simulink model "cart_pole_model"  (R2020b)
settings: Solver=VariableStepAuto  StartTime=0.0  StopTime=10.0  RelTol=1e-3
undefined symbols (not defined in the file): b, D_theta, D_x, g, I, I_theta, I_x, l, m, M, P_theta, P_x
libraries: pid_lib x4
settings Model: Creator=Illia  LastModifiedBy=Illia

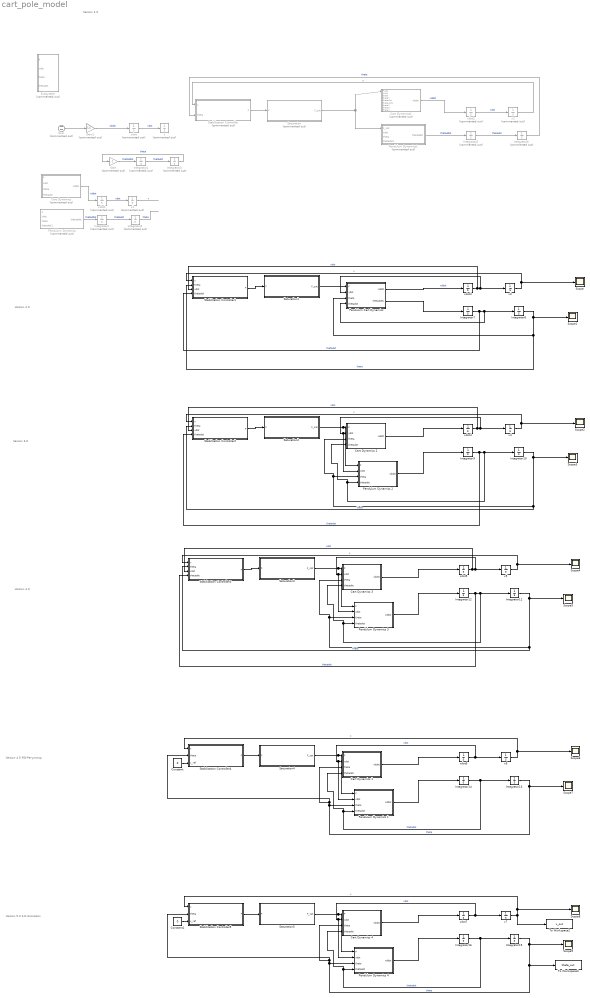
== system cart_pole_model ==
  note: Version 1.0
  note: Version 2.0
  note: Version 3.0
  note: Version 4.0
  note: Version 4.5
      | PID-Регулятор
  note: Version 5.0
      | 2-D Animation
  Cart Dynamics : Subsystem  Commented=on
  Cart Dynamics 1 : Subsystem
  Cart Dynamics 2 : Subsystem
  Cart Dynamics 3 : Subsystem
  Cart Dynamics 4 : Subsystem
  Cart Dynamics1 : Subsystem  Commented=on
  Constant : Constant  Value=0
  Constant1 : Constant  Value=0
  Gain : Gain  Commented=on  Gain=-1
  Gain1 : Gain  Commented=on  Gain=50
  Integrator{1..5} (5 alike) : Integrator  Commented=on
  Integrator{8,10..11,13,15} (5 alike) : Integrator  InitialCondition=0.1
  Integrator{7,9,12,14,16} (5 alike) : Integrator
  Integrator6 : Integrator  Commented=on  InitialCondition=0.1
  Pendulum Cart Dynamics : MATLAB Function  TreatAsAtomicUnit=on
  Pendulum Dynamics : Subsystem  Commented=on
  Pendulum Dynamics 1 : Subsystem
  Pendulum Dynamics 2 : Subsystem
  Pendulum Dynamics 3 : Subsystem
  Pendulum Dynamics 4 : Subsystem
  Pendulum Dynamics1 : Subsystem  Commented=on
  Saturation : Subsystem  Commented=on
  Saturation1 : Subsystem
  Saturation2 : Subsystem
  Saturation3 : Subsystem
  Saturation4 : Subsystem
  Saturation5 : Subsystem
  Scope{,1..9} (10 alike) : Scope
  Stabilization Controller : Subsystem  Commented=on
  Stabilization Controller1 : Subsystem
  Stabilization Controller2 : Subsystem
  Stabilization Controller3 : Subsystem
  Stabilization Controller4 : Subsystem
  Stabilization Controller5 : Subsystem
  Subsystem : Subsystem  Commented=on
  Sum : Sum  Commented=on  Inputs=--
  To Workspace2 : ToWorkspace  VariableName=x_out  SampleTime=-1
      settings: Save2DSignal=2-D array (concatenate along first dimension)
  To Workspace3 : ToWorkspace  VariableName=theta_out  SampleTime=-1
      settings: Save2DSignal=2-D array (concatenate along first dimension)
  x : Integrator  Commented=on
  x1 : Integrator  Commented=on
  x2 : Integrator  Commented=on
  x{3..7} (5 alike) : Integrator
  xdot : Integrator  Commented=on
  xdot1 : Integrator  Commented=on
  xdot2 : Integrator  Commented=on
  xdot{3..7} (5 alike) : Integrator
  wires:
  xdot/1 -> x/1  "xdot"
  Gain/1 -> Integrator1/1  "thetaddot"
  Integrator1/1 -> Integrator3/1  "thetadot"
  ? -> Sum/2  "theta"
  ? -> Sum/1  "x"
  Sum/1 -> Gain1/1
  Gain1/1 -> xdot/1  "xddot"
  Integrator3/1 -> Gain/1  "theta"
  Stabilization Controller/1(F) -> Saturation/1(F)
  Saturation/1(F_sat) -> Cart Dynamics1/1(F_sat), Pendulum Dynamics1/1(F_sat)
  Pendulum Dynamics1/1(thetaddot) -> Integrator5/1  "thetaddot"
  xdot2/1 -> x2/1  "xdot"
  Cart Dynamics1/1(xddot) -> xdot2/1  "xddot"
  Pendulum Dynamics/1(thetaddot) -> Integrator2/1  "thetaddot"
  Integrator2/1 -> Integrator4/1  "thetadot"
  Integrator4/1 -> ?  "theta"
  x1/1 -> ?  "x"
  xdot1/1 -> x1/1  "xdot"
  Cart Dynamics/1(xddot) -> xdot1/1  "xddot"
  Integrator5/1 -> Integrator6/1  "thetadot"
  Integrator6/1 -> Stabilization Controller/2(theta)  "theta"
  x2/1 -> Stabilization Controller/1(x)  "x"
  x3/1 -> Scope/1, Stabilization Controller1/1(x)  "x"
  xdot3/1 -> Stabilization Controller1/3(xdot), Pendulum Cart Dynamics/2(xdot), x3/1  "xdot"
  Stabilization Controller1/1(F) -> Saturation1/1(F)
  Integrator8/1 -> Scope1/1, Pendulum Cart Dynamics/3(theta), Stabilization Controller1/2(theta)  "theta"
  Pendulum Cart Dynamics/1(xddot) -> xdot3/1  "xddot"
  Saturation1/1(F_sat) -> Pendulum Cart Dynamics/1(F)
  Integrator7/1 -> Stabilization Controller1/4(thetadot), Pendulum Cart Dynamics/4(thetadot), Integrator8/1  "thetadot"
  Pendulum Cart Dynamics/2(thetaddot) -> Integrator7/1
  Stabilization Controller2/1(F) -> Saturation2/1(F)
  Integrator9/1 -> Stabilization Controller2/4(thetadot), Cart Dynamics 2/4(thetadot), Pendulum Dynamics 2/4(thetadot), Integrator10/1  "thetadot"
  xdot4/1 -> Stabilization Controller2/3(xdot), Pendulum Dynamics 2/2(xdot), Cart Dynamics 2/2(xdot), x4/1  "xdot"
  Integrator10/1 -> Scope3/1, Cart Dynamics 2/3(theta), Pendulum Dynamics 2/3(theta), Stabilization Controller2/2(theta)  "theta"
  x4/1 -> Scope2/1, Stabilization Controller2/1(x)  "x"
  Saturation2/1(F_sat) -> Pendulum Dynamics 2/1(F), Cart Dynamics 2/1(F)
  Cart Dynamics 2/1(xddot) -> xdot4/1
  Pendulum Dynamics 2/1(xddot) -> Integrator9/1
  Pendulum Dynamics 3/1(xddot) -> Integrator12/1
  Stabilization Controller3/1(F) -> Saturation3/1(F)
  x5/1 -> Scope4/1, Stabilization Controller3/1(x)  "x"
  Saturation3/1(F_sat) -> Pendulum Dynamics 3/1(F), Cart Dynamics 3/1(F)
  xdot5/1 -> Stabilization Controller3/3(xdot), Pendulum Dynamics 3/2(xdot), Cart Dynamics 3/2(xdot), x5/1  "xdot"
  Integrator12/1 -> Stabilization Controller3/4(thetadot), Cart Dynamics 3/4(thetadot), Pendulum Dynamics 3/4(thetadot), Integrator11/1  "thetadot"
  Cart Dynamics 3/1(xddot) -> xdot5/1
  Integrator11/1 -> Scope5/1, Cart Dynamics 3/3(theta), Pendulum Dynamics 3/3(theta), Stabilization Controller3/2(theta)  "theta"
  Integrator14/1 -> Cart Dynamics 1/4(thetadot), Pendulum Dynamics 1/4(thetadot), Integrator13/1  "thetadot"
  Integrator13/1 -> Scope7/1, Stabilization Controller4/2(theta), Cart Dynamics 1/3(theta), Pendulum Dynamics 1/3(theta)  "theta"
  xdot6/1 -> Pendulum Dynamics 1/2(xdot), Cart Dynamics 1/2(xdot), x6/1  "xdot"
  Saturation4/1(F_sat) -> Pendulum Dynamics 1/1(F), Cart Dynamics 1/1(F)
  x6/1 -> Scope6/1, Stabilization Controller4/1(x)  "x"
  Stabilization Controller4/1(F) -> Saturation4/1(F)
  Cart Dynamics 1/1(xddot) -> xdot6/1
  Pendulum Dynamics 1/1(xddot) -> Integrator14/1
  Constant/1 -> Stabilization Controller4/3(x_ref)
  Integrator16/1 -> Cart Dynamics 4/4(thetadot), Pendulum Dynamics 4/4(thetadot), Integrator15/1  "thetadot"
  Cart Dynamics 4/1(xddot) -> xdot7/1
  Pendulum Dynamics 4/1(xddot) -> Integrator16/1
  Stabilization Controller5/1(F) -> Saturation5/1(F)
  Constant1/1 -> Stabilization Controller5/3(x_ref)
  x7/1 -> Scope8/1, Stabilization Controller5/1(x), To Workspace2/1  "x"
  Saturation5/1(F_sat) -> Pendulum Dynamics 4/1(F), Cart Dynamics 4/1(F)
  xdot7/1 -> Pendulum Dynamics 4/2(xdot), Cart Dynamics 4/2(xdot), x7/1  "xdot"
  Integrator15/1 -> Scope9/1, To Workspace3/1, Stabilization Controller5/2(theta), Cart Dynamics 4/3(theta), Pendulum Dynamics 4/3(theta)  "theta"

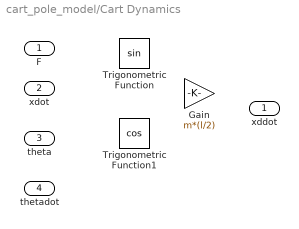
== system cart_pole_model/Cart Dynamics ==
  F : Inport
  xdot : Inport  Port=2
  theta : Inport  Port=3
  thetadot : Inport  Port=4
  Gain : Gain  Gain=m*(l/2)
  Trigonometric Function : Trigonometry
  Trigonometric Function1 : Trigonometry  Operator=cos
  xddot : Outport

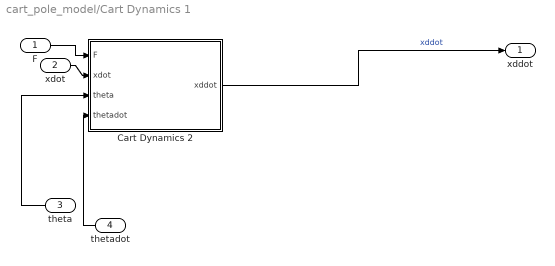
== system cart_pole_model/Cart Dynamics 1 ==
  F : Inport
  xdot : Inport  Port=2
  theta : Inport  Port=3
  thetadot : Inport  Port=4
  Cart Dynamics 2 : MATLAB Function  TreatAsAtomicUnit=on
  xddot : Outport
  wires:
  xdot/1 -> Cart Dynamics 2/2(xdot)
  thetadot/1 -> Cart Dynamics 2/4(thetadot)
  Cart Dynamics 2/1(xddot) -> xddot/1  "xddot"
  F/1 -> Cart Dynamics 2/1(F)
  theta/1 -> Cart Dynamics 2/3(theta)

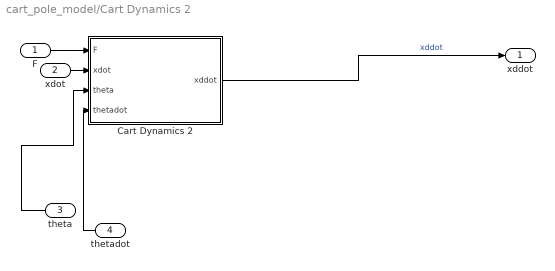
== system cart_pole_model/Cart Dynamics 2 ==
  F : Inport
  xdot : Inport  Port=2
  theta : Inport  Port=3
  thetadot : Inport  Port=4
  Cart Dynamics 2 : MATLAB Function  TreatAsAtomicUnit=on
  xddot : Outport
  wires:
  xdot/1 -> Cart Dynamics 2/2(xdot)
  thetadot/1 -> Cart Dynamics 2/4(thetadot)
  Cart Dynamics 2/1(xddot) -> xddot/1  "xddot"
  F/1 -> Cart Dynamics 2/1(F)
  theta/1 -> Cart Dynamics 2/3(theta)

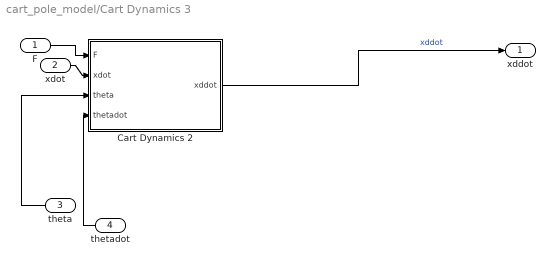
== system cart_pole_model/Cart Dynamics 3 ==
  F : Inport
  xdot : Inport  Port=2
  theta : Inport  Port=3
  thetadot : Inport  Port=4
  Cart Dynamics 2 : MATLAB Function  TreatAsAtomicUnit=on
  xddot : Outport
  wires:
  xdot/1 -> Cart Dynamics 2/2(xdot)
  thetadot/1 -> Cart Dynamics 2/4(thetadot)
  Cart Dynamics 2/1(xddot) -> xddot/1  "xddot"
  F/1 -> Cart Dynamics 2/1(F)
  theta/1 -> Cart Dynamics 2/3(theta)

== system cart_pole_model/Cart Dynamics 4 ==
  F : Inport
  xdot : Inport  Port=2
  theta : Inport  Port=3
  thetadot : Inport  Port=4
  Cart Dynamics 2 : MATLAB Function  TreatAsAtomicUnit=on
  xddot : Outport
  wires:
  xdot/1 -> Cart Dynamics 2/2(xdot)
  thetadot/1 -> Cart Dynamics 2/4(thetadot)
  Cart Dynamics 2/1(xddot) -> xddot/1  "xddot"
  F/1 -> Cart Dynamics 2/1(F)
  theta/1 -> Cart Dynamics 2/3(theta)

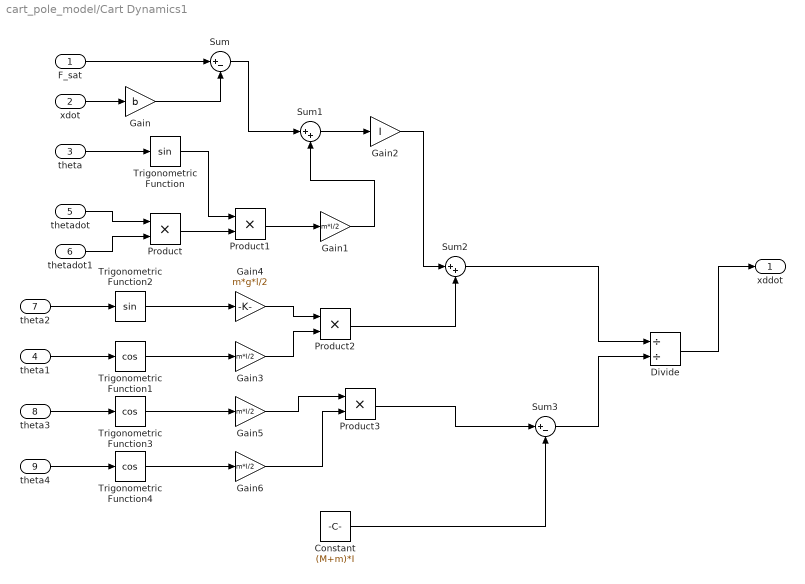
== system cart_pole_model/Cart Dynamics1 ==
  F_sat : Inport
  xdot : Inport  Port=2
  theta : Inport  Port=3
  theta1 : Inport  Port=4
  thetadot : Inport  Port=5
  thetadot1 : Inport  Port=6
  theta2 : Inport  Port=7
  theta3 : Inport  Port=8
  theta4 : Inport  Port=9
  Constant : Constant  Value=(M+m)*I
  Divide : Product  Inputs=//
  Gain : Gain  Gain=b
  Gain{1,3,5..6} (4 alike) : Gain  Gain=m*l/2
  Gain2 : Gain  Gain=I
  Gain4 : Gain  Gain=m*g*l/2
  Product{,1..3} (4 alike) : Product
  Sum : Sum  Inputs=|+-
  Sum1 : Sum  Inputs=|++
  Sum2 : Sum  Inputs=|++
  Sum3 : Sum  Inputs=|+-
  Trigonometric Function : Trigonometry
  Trigonometric Function1 : Trigonometry  Operator=cos
  Trigonometric Function2 : Trigonometry
  Trigonometric Function3 : Trigonometry  Operator=cos
  Trigonometric Function4 : Trigonometry  Operator=cos
  xddot : Outport
  wires:
  theta/1 -> Trigonometric Function/1
  theta1/1 -> Trigonometric Function1/1
  xdot/1 -> Gain/1
  F_sat/1 -> Sum/1
  Gain/1 -> Sum/2
  thetadot/1 -> Product/1
  thetadot1/1 -> Product/2
  Trigonometric Function/1 -> Product1/1
  Product/1 -> Product1/2
  Product1/1 -> Gain1/1
  Sum/1 -> Sum1/1
  Gain1/1 -> Sum1/2
  Sum1/1 -> Gain2/1
  Trigonometric Function1/1 -> Gain3/1
  theta2/1 -> Trigonometric Function2/1
  Trigonometric Function2/1 -> Gain4/1
  Gain4/1 -> Product2/1
  Gain3/1 -> Product2/2
  Gain2/1 -> Sum2/1
  Product2/1 -> Sum2/2
  Trigonometric Function3/1 -> Gain5/1
  theta3/1 -> Trigonometric Function3/1
  Gain5/1 -> Product3/1
  theta4/1 -> Trigonometric Function4/1
  Trigonometric Function4/1 -> Gain6/1
  Gain6/1 -> Product3/2
  Constant/1 -> Sum3/2
  Product3/1 -> Sum3/1
  Divide/1 -> xddot/1
  Sum3/1 -> Divide/2
  Sum2/1 -> Divide/1

== system cart_pole_model/Pendulum Dynamics ==
  F : Inport
  xdot : Inport  Port=2
  theta : Inport  Port=3
  thetadot1 : Inport  Port=4
  thetaddot : Outport

== system cart_pole_model/Pendulum Dynamics 1 ==
  F : Inport
  xdot : Inport  Port=2
  theta : Inport  Port=3
  thetadot : Inport  Port=4
  Pendulum Dynamics 2 : MATLAB Function  TreatAsAtomicUnit=on
  xddot : Outport
  wires:
  xdot/1 -> Pendulum Dynamics 2/2(xdot)
  F/1 -> Pendulum Dynamics 2/1(F)
  Pendulum Dynamics 2/1(thetaddot) -> xddot/1  "xddot"
  thetadot/1 -> Pendulum Dynamics 2/4(thetadot)
  theta/1 -> Pendulum Dynamics 2/3(theta)

== system cart_pole_model/Pendulum Dynamics 2 ==
  F : Inport
  xdot : Inport  Port=2
  theta : Inport  Port=3
  thetadot : Inport  Port=4
  Pendulum Dynamics 2 : MATLAB Function  TreatAsAtomicUnit=on
  xddot : Outport
  wires:
  xdot/1 -> Pendulum Dynamics 2/2(xdot)
  F/1 -> Pendulum Dynamics 2/1(F)
  Pendulum Dynamics 2/1(thetaddot) -> xddot/1  "xddot"
  thetadot/1 -> Pendulum Dynamics 2/4(thetadot)
  theta/1 -> Pendulum Dynamics 2/3(theta)

== system cart_pole_model/Pendulum Dynamics 3 ==
  F : Inport
  xdot : Inport  Port=2
  theta : Inport  Port=3
  thetadot : Inport  Port=4
  Pendulum Dynamics 2 : MATLAB Function  TreatAsAtomicUnit=on
  xddot : Outport
  wires:
  xdot/1 -> Pendulum Dynamics 2/2(xdot)
  F/1 -> Pendulum Dynamics 2/1(F)
  Pendulum Dynamics 2/1(thetaddot) -> xddot/1  "xddot"
  thetadot/1 -> Pendulum Dynamics 2/4(thetadot)
  theta/1 -> Pendulum Dynamics 2/3(theta)

== system cart_pole_model/Pendulum Dynamics 4 ==
  F : Inport
  xdot : Inport  Port=2
  theta : Inport  Port=3
  thetadot : Inport  Port=4
  Pendulum Dynamics 2 : MATLAB Function  TreatAsAtomicUnit=on
  xddot : Outport
  wires:
  xdot/1 -> Pendulum Dynamics 2/2(xdot)
  F/1 -> Pendulum Dynamics 2/1(F)
  Pendulum Dynamics 2/1(thetaddot) -> xddot/1  "xddot"
  thetadot/1 -> Pendulum Dynamics 2/4(thetadot)
  theta/1 -> Pendulum Dynamics 2/3(theta)

== system cart_pole_model/Pendulum Dynamics1 ==
  F_sat : Inport
  xdot : Inport  Port=2
  theta : Inport  Port=3
  thetadot1 : Inport  Port=4
  Gain : Gain  Gain=-1
  thetaddot : Outport
  wires:
  theta/1 -> Gain/1
  Gain/1 -> thetaddot/1

== system cart_pole_model/Saturation ==
  F : Inport
  Saturation : Saturate
  F_sat : Outport
  wires:
  F/1 -> Saturation/1
  Saturation/1 -> F_sat/1

== system cart_pole_model/Saturation1 ==
  F : Inport
  Saturation : Saturate
  F_sat : Outport
  wires:
  F/1 -> Saturation/1
  Saturation/1 -> F_sat/1

== system cart_pole_model/Saturation2 ==
  F : Inport
  Saturation : Saturate
  F_sat : Outport
  wires:
  F/1 -> Saturation/1
  Saturation/1 -> F_sat/1

== system cart_pole_model/Saturation3 ==
  F : Inport
  Saturation : Saturate
  F_sat : Outport
  wires:
  F/1 -> Saturation/1
  Saturation/1 -> F_sat/1

== system cart_pole_model/Saturation4 ==
  F : Inport
  Saturation : Saturate
  F_sat : Outport
  wires:
  F/1 -> Saturation/1
  Saturation/1 -> F_sat/1

== system cart_pole_model/Saturation5 ==
  F : Inport
  Saturation : Saturate
  F_sat : Outport
  wires:
  F/1 -> Saturation/1
  Saturation/1 -> F_sat/1

== system cart_pole_model/Stabilization Controller ==
  x : Inport
  theta : Inport  Port=2
  Gain1 : Gain  Gain=-10
  Gain2 : Gain  Gain=-1
  Sum : Sum  Inputs=|++
  F : Outport
  wires:
  x/1 -> Gain2/1
  theta/1 -> Gain1/1
  Sum/1 -> F/1
  Gain1/1 -> Sum/2
  Gain2/1 -> Sum/1

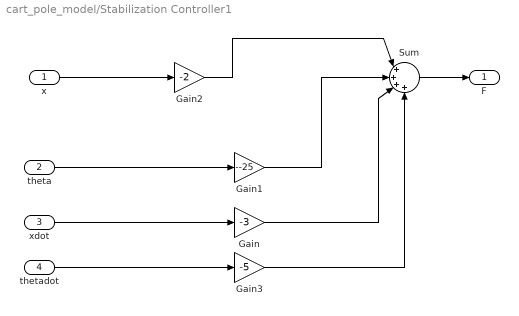
== system cart_pole_model/Stabilization Controller1 ==
  x : Inport
  theta : Inport  Port=2
  xdot : Inport  Port=3
  thetadot : Inport  Port=4
  Gain : Gain  Gain=-3
  Gain1 : Gain  Gain=--25
  Gain2 : Gain  Gain=-2
  Gain3 : Gain  Gain=-5
  Sum : Sum  Inputs=|++++
  F : Outport
  wires:
  x/1 -> Gain2/1
  theta/1 -> Gain1/1
  Sum/1 -> F/1
  Gain1/1 -> Sum/2
  Gain2/1 -> Sum/1
  xdot/1 -> Gain/1
  thetadot/1 -> Gain3/1
  Gain/1 -> Sum/3
  Gain3/1 -> Sum/4

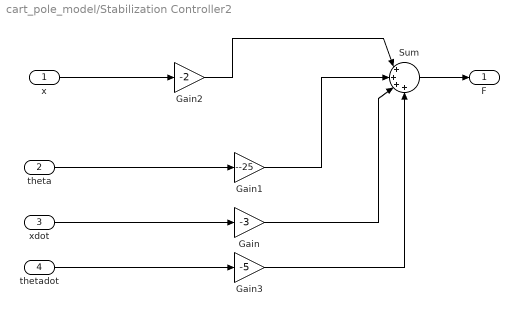
== system cart_pole_model/Stabilization Controller2 ==
  x : Inport
  theta : Inport  Port=2
  xdot : Inport  Port=3
  thetadot : Inport  Port=4
  Gain : Gain  Gain=-3
  Gain1 : Gain  Gain=--25
  Gain2 : Gain  Gain=-2
  Gain3 : Gain  Gain=-5
  Sum : Sum  Inputs=|++++
  F : Outport
  wires:
  x/1 -> Gain2/1
  theta/1 -> Gain1/1
  Sum/1 -> F/1
  Gain1/1 -> Sum/2
  Gain2/1 -> Sum/1
  xdot/1 -> Gain/1
  thetadot/1 -> Gain3/1
  Gain/1 -> Sum/3
  Gain3/1 -> Sum/4

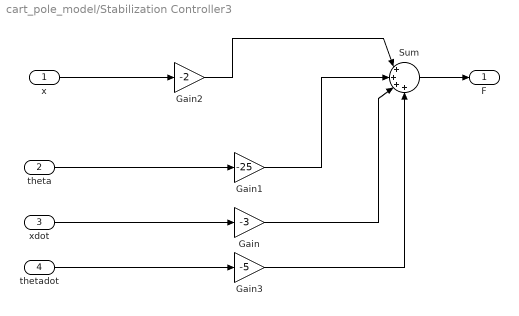
== system cart_pole_model/Stabilization Controller3 ==
  x : Inport
  theta : Inport  Port=2
  xdot : Inport  Port=3
  thetadot : Inport  Port=4
  Gain : Gain  Gain=-3
  Gain1 : Gain  Gain=-25
  Gain2 : Gain  Gain=-2
  Gain3 : Gain  Gain=-5
  Sum : Sum  Inputs=|++++
  F : Outport
  wires:
  x/1 -> Gain2/1
  theta/1 -> Gain1/1
  Sum/1 -> F/1
  Gain1/1 -> Sum/2
  Gain2/1 -> Sum/1
  xdot/1 -> Gain/1
  thetadot/1 -> Gain3/1
  Gain/1 -> Sum/3
  Gain3/1 -> Sum/4

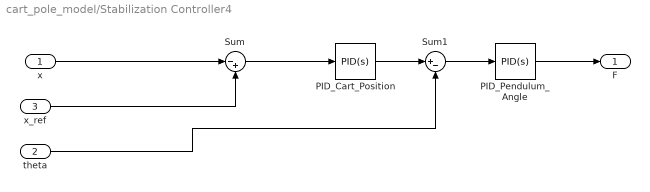
== system cart_pole_model/Stabilization Controller4 ==
  x : Inport
  theta : Inport  Port=2
  x_ref : Inport  Port=3
  PID_Cart_Position : pid_lib/PID Controller  Controller=PID  Form=Parallel  TimeDomain=Continuous-time  UseExternalTs=off  SampleTime=-1  IntegratorMethod=Forward Euler  FilterMethod=Forward Euler  ControllerParametersSource=internal  P=P_x  I=I_x  D=D_x  UseFilter=on  N=100  TunerSelectOption=Transfer Function Based (PID Tuner App)  InitialConditionSource=internal  InitialConditionForIntegrator=0  InitialConditionForFilter=0  DifferentiatorICPrevScaledInput=0  ExternalReset=none  TrackingMode=off  Kt=1  LimitOutput=off  SatLimitsSource=internal  UpperSaturationLimit=inf  LowerSaturationLimit=-inf  LinearizeAsGain=on  AntiWindupMode=none  Kb=1  POutMin=[]  POutMax=[]  IOutMin=[]  IOutMax=[]  DOutMin=[]  DOutMax=[]  NOutMin=[]  NOutMax=[]  SumOutMin=[]  SumOutMax=[]  SaturationOutMin=[]  SaturationOutMax=[]  PParamMin=[]  PParamMax=[]  IParamMin=[]  IParamMax=[]  DParamMin=[]  DParamMax=[]  NParamMin=[]  NParamMax=[]  KbParamMin=[]  KbParamMax=[]  KtParamMin=[]  KtParamMax=[]  KbOutMin=[]  KbOutMax=[]  KtOutMin=[]  KtOutMax=[]  IntegratorOutMin=[]  IntegratorOutMax=[]  FilterOutMin=[]  FilterOutMax=[]  SumI1OutMin=[]  SumI1OutMax=[]  SumI2OutMin=[]  SumI2OutMax=[]  SumI3OutMin=[]  SumI3OutMax=[]  SumI4OutMin=[]  SumI4OutMax=[]  SumDOutMin=[]  SumDOutMax=[]  DifferentiatorOutMin=[]  DifferentiatorOutMax=[]  FilterDiffOutCoefMin=[]  FilterDiffOutCoefMax=[]  ReciprocalOutMin=[]  ReciprocalOutMax=[]  SumDenOutMin=[]  SumDenOutMax=[]  SumNumOutMin=[]  SumNumOutMax=[]  DivideOutMin=[]  DivideOutMax=[]  UdiffTsProdOutMin=[]  UdiffTsProdOutMax=[]  NTsProdOutMin=[]  NTsProdOutMax=[]  UintegralTsProdOutMin=[]  UintegralTsProdOutMax=[]  UngainTsProdOutMin=[]  UngainTsProdOutMax=[]  IntegratorContinuousStateAttributes=''  IntegratorStateMustResolveToSignalObject=off  IntegratorRTWStateStorageClass=Auto  FilterContinuousStateAttributes=''  FilterStateMustResolveToSignalObject=off  FilterRTWStateStorageClass=Auto  ParallelPVariant=InternalParameters  IdealPVariant=Disabled  IVariant=InternalParameters  DVariant=InternalParameters  IntegratorVariant=Continuous  SatVariant=Disabled  AWVariant=Passthrough  PCopyVariant=Disabled  TRVariant=Disabled  FdbkBlocksVariant=Forward  IdealPFdbkVariant=Disabled  SatFdbkVariant=Disabled  DerivativeFilterVariant=ContFilter  NVariant=InternalParameters  NCopyVariant=Disabled  FilterICVariant=InternalICsFilter  IntegratorICVariant=InternalICs  ExternalResetVariant=Disabled  TRSumVariant=Passthrough  SumFdbkVariant=Disabled  SumVariant=Sum_PID  TsampFilterVariant=InternalTs  TsampNgainVariant=Passthrough  TsampIntegralVariant=Passthrough  ExternalSaturationOutDataTypeStr=Inherit: Same as second input
  PID_Pendulum_Angle : pid_lib/PID Controller  Controller=PID  Form=Parallel  TimeDomain=Continuous-time  UseExternalTs=off  SampleTime=-1  IntegratorMethod=Forward Euler  FilterMethod=Forward Euler  ControllerParametersSource=internal  P=P_theta  I=I_theta  D=D_theta  UseFilter=on  N=100  TunerSelectOption=Transfer Function Based (PID Tuner App)  InitialConditionSource=internal  InitialConditionForIntegrator=0  InitialConditionForFilter=0  DifferentiatorICPrevScaledInput=0  ExternalReset=none  TrackingMode=off  Kt=1  LimitOutput=off  SatLimitsSource=internal  UpperSaturationLimit=inf  LowerSaturationLimit=-inf  LinearizeAsGain=on  AntiWindupMode=none  Kb=1  POutMin=[]  POutMax=[]  IOutMin=[]  IOutMax=[]  DOutMin=[]  DOutMax=[]  NOutMin=[]  NOutMax=[]  SumOutMin=[]  SumOutMax=[]  SaturationOutMin=[]  SaturationOutMax=[]  PParamMin=[]  PParamMax=[]  IParamMin=[]  IParamMax=[]  DParamMin=[]  DParamMax=[]  NParamMin=[]  NParamMax=[]  KbParamMin=[]  KbParamMax=[]  KtParamMin=[]  KtParamMax=[]  KbOutMin=[]  KbOutMax=[]  KtOutMin=[]  KtOutMax=[]  IntegratorOutMin=[]  IntegratorOutMax=[]  FilterOutMin=[]  FilterOutMax=[]  SumI1OutMin=[]  SumI1OutMax=[]  SumI2OutMin=[]  SumI2OutMax=[]  SumI3OutMin=[]  SumI3OutMax=[]  SumI4OutMin=[]  SumI4OutMax=[]  SumDOutMin=[]  SumDOutMax=[]  DifferentiatorOutMin=[]  DifferentiatorOutMax=[]  FilterDiffOutCoefMin=[]  FilterDiffOutCoefMax=[]  ReciprocalOutMin=[]  ReciprocalOutMax=[]  SumDenOutMin=[]  SumDenOutMax=[]  SumNumOutMin=[]  SumNumOutMax=[]  DivideOutMin=[]  DivideOutMax=[]  UdiffTsProdOutMin=[]  UdiffTsProdOutMax=[]  NTsProdOutMin=[]  NTsProdOutMax=[]  UintegralTsProdOutMin=[]  UintegralTsProdOutMax=[]  UngainTsProdOutMin=[]  UngainTsProdOutMax=[]  IntegratorContinuousStateAttributes=''  IntegratorStateMustResolveToSignalObject=off  IntegratorRTWStateStorageClass=Auto  FilterContinuousStateAttributes=''  FilterStateMustResolveToSignalObject=off  FilterRTWStateStorageClass=Auto  ParallelPVariant=InternalParameters  IdealPVariant=Disabled  IVariant=InternalParameters  DVariant=InternalParameters  IntegratorVariant=Continuous  SatVariant=Disabled  AWVariant=Passthrough  PCopyVariant=Disabled  TRVariant=Disabled  FdbkBlocksVariant=Forward  IdealPFdbkVariant=Disabled  SatFdbkVariant=Disabled  DerivativeFilterVariant=ContFilter  NVariant=InternalParameters  NCopyVariant=Disabled  FilterICVariant=InternalICsFilter  IntegratorICVariant=InternalICs  ExternalResetVariant=Disabled  TRSumVariant=Passthrough  SumFdbkVariant=Disabled  SumVariant=Sum_PID  TsampFilterVariant=InternalTs  TsampNgainVariant=Passthrough  TsampIntegralVariant=Passthrough  ExternalSaturationOutDataTypeStr=Inherit: Same as second input
  Sum : Sum  Inputs=|-+
  Sum1 : Sum  Inputs=|+-
  F : Outport
  wires:
  x/1 -> Sum/1
  x_ref/1 -> Sum/2
  Sum/1 -> PID_Cart_Position/1
  PID_Cart_Position/1 -> Sum1/1
  theta/1 -> Sum1/2
  Sum1/1 -> PID_Pendulum_Angle/1
  PID_Pendulum_Angle/1 -> F/1

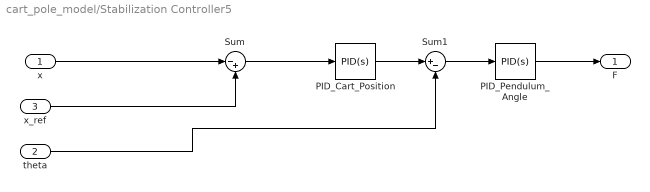
== system cart_pole_model/Stabilization Controller5 ==
  x : Inport
  theta : Inport  Port=2
  x_ref : Inport  Port=3
  PID_Cart_Position : pid_lib/PID Controller  Controller=PID  Form=Parallel  TimeDomain=Continuous-time  UseExternalTs=off  SampleTime=-1  IntegratorMethod=Forward Euler  FilterMethod=Forward Euler  ControllerParametersSource=internal  P=P_x  I=I_x  D=D_x  UseFilter=on  N=100  TunerSelectOption=Transfer Function Based (PID Tuner App)  InitialConditionSource=internal  InitialConditionForIntegrator=0  InitialConditionForFilter=0  DifferentiatorICPrevScaledInput=0  ExternalReset=none  TrackingMode=off  Kt=1  LimitOutput=off  SatLimitsSource=internal  UpperSaturationLimit=inf  LowerSaturationLimit=-inf  LinearizeAsGain=on  AntiWindupMode=none  Kb=1  POutMin=[]  POutMax=[]  IOutMin=[]  IOutMax=[]  DOutMin=[]  DOutMax=[]  NOutMin=[]  NOutMax=[]  SumOutMin=[]  SumOutMax=[]  SaturationOutMin=[]  SaturationOutMax=[]  PParamMin=[]  PParamMax=[]  IParamMin=[]  IParamMax=[]  DParamMin=[]  DParamMax=[]  NParamMin=[]  NParamMax=[]  KbParamMin=[]  KbParamMax=[]  KtParamMin=[]  KtParamMax=[]  KbOutMin=[]  KbOutMax=[]  KtOutMin=[]  KtOutMax=[]  IntegratorOutMin=[]  IntegratorOutMax=[]  FilterOutMin=[]  FilterOutMax=[]  SumI1OutMin=[]  SumI1OutMax=[]  SumI2OutMin=[]  SumI2OutMax=[]  SumI3OutMin=[]  SumI3OutMax=[]  SumI4OutMin=[]  SumI4OutMax=[]  SumDOutMin=[]  SumDOutMax=[]  DifferentiatorOutMin=[]  DifferentiatorOutMax=[]  FilterDiffOutCoefMin=[]  FilterDiffOutCoefMax=[]  ReciprocalOutMin=[]  ReciprocalOutMax=[]  SumDenOutMin=[]  SumDenOutMax=[]  SumNumOutMin=[]  SumNumOutMax=[]  DivideOutMin=[]  DivideOutMax=[]  UdiffTsProdOutMin=[]  UdiffTsProdOutMax=[]  NTsProdOutMin=[]  NTsProdOutMax=[]  UintegralTsProdOutMin=[]  UintegralTsProdOutMax=[]  UngainTsProdOutMin=[]  UngainTsProdOutMax=[]  IntegratorContinuousStateAttributes=''  IntegratorStateMustResolveToSignalObject=off  IntegratorRTWStateStorageClass=Auto  FilterContinuousStateAttributes=''  FilterStateMustResolveToSignalObject=off  FilterRTWStateStorageClass=Auto  ParallelPVariant=InternalParameters  IdealPVariant=Disabled  IVariant=InternalParameters  DVariant=InternalParameters  IntegratorVariant=Continuous  SatVariant=Disabled  AWVariant=Passthrough  PCopyVariant=Disabled  TRVariant=Disabled  FdbkBlocksVariant=Forward  IdealPFdbkVariant=Disabled  SatFdbkVariant=Disabled  DerivativeFilterVariant=ContFilter  NVariant=InternalParameters  NCopyVariant=Disabled  FilterICVariant=InternalICsFilter  IntegratorICVariant=InternalICs  ExternalResetVariant=Disabled  TRSumVariant=Passthrough  SumFdbkVariant=Disabled  SumVariant=Sum_PID  TsampFilterVariant=InternalTs  TsampNgainVariant=Passthrough  TsampIntegralVariant=Passthrough  ExternalSaturationOutDataTypeStr=Inherit: Same as second input
  PID_Pendulum_Angle : pid_lib/PID Controller  Controller=PID  Form=Parallel  TimeDomain=Continuous-time  UseExternalTs=off  SampleTime=-1  IntegratorMethod=Forward Euler  FilterMethod=Forward Euler  ControllerParametersSource=internal  P=P_theta  I=I_theta  D=D_theta  UseFilter=on  N=100  TunerSelectOption=Transfer Function Based (PID Tuner App)  InitialConditionSource=internal  InitialConditionForIntegrator=0  InitialConditionForFilter=0  DifferentiatorICPrevScaledInput=0  ExternalReset=none  TrackingMode=off  Kt=1  LimitOutput=off  SatLimitsSource=internal  UpperSaturationLimit=inf  LowerSaturationLimit=-inf  LinearizeAsGain=on  AntiWindupMode=none  Kb=1  POutMin=[]  POutMax=[]  IOutMin=[]  IOutMax=[]  DOutMin=[]  DOutMax=[]  NOutMin=[]  NOutMax=[]  SumOutMin=[]  SumOutMax=[]  SaturationOutMin=[]  SaturationOutMax=[]  PParamMin=[]  PParamMax=[]  IParamMin=[]  IParamMax=[]  DParamMin=[]  DParamMax=[]  NParamMin=[]  NParamMax=[]  KbParamMin=[]  KbParamMax=[]  KtParamMin=[]  KtParamMax=[]  KbOutMin=[]  KbOutMax=[]  KtOutMin=[]  KtOutMax=[]  IntegratorOutMin=[]  IntegratorOutMax=[]  FilterOutMin=[]  FilterOutMax=[]  SumI1OutMin=[]  SumI1OutMax=[]  SumI2OutMin=[]  SumI2OutMax=[]  SumI3OutMin=[]  SumI3OutMax=[]  SumI4OutMin=[]  SumI4OutMax=[]  SumDOutMin=[]  SumDOutMax=[]  DifferentiatorOutMin=[]  DifferentiatorOutMax=[]  FilterDiffOutCoefMin=[]  FilterDiffOutCoefMax=[]  ReciprocalOutMin=[]  ReciprocalOutMax=[]  SumDenOutMin=[]  SumDenOutMax=[]  SumNumOutMin=[]  SumNumOutMax=[]  DivideOutMin=[]  DivideOutMax=[]  UdiffTsProdOutMin=[]  UdiffTsProdOutMax=[]  NTsProdOutMin=[]  NTsProdOutMax=[]  UintegralTsProdOutMin=[]  UintegralTsProdOutMax=[]  UngainTsProdOutMin=[]  UngainTsProdOutMax=[]  IntegratorContinuousStateAttributes=''  IntegratorStateMustResolveToSignalObject=off  IntegratorRTWStateStorageClass=Auto  FilterContinuousStateAttributes=''  FilterStateMustResolveToSignalObject=off  FilterRTWStateStorageClass=Auto  ParallelPVariant=InternalParameters  IdealPVariant=Disabled  IVariant=InternalParameters  DVariant=InternalParameters  IntegratorVariant=Continuous  SatVariant=Disabled  AWVariant=Passthrough  PCopyVariant=Disabled  TRVariant=Disabled  FdbkBlocksVariant=Forward  IdealPFdbkVariant=Disabled  SatFdbkVariant=Disabled  DerivativeFilterVariant=ContFilter  NVariant=InternalParameters  NCopyVariant=Disabled  FilterICVariant=InternalICsFilter  IntegratorICVariant=InternalICs  ExternalResetVariant=Disabled  TRSumVariant=Passthrough  SumFdbkVariant=Disabled  SumVariant=Sum_PID  TsampFilterVariant=InternalTs  TsampNgainVariant=Passthrough  TsampIntegralVariant=Passthrough  ExternalSaturationOutDataTypeStr=Inherit: Same as second input
  Sum : Sum  Inputs=|-+
  Sum1 : Sum  Inputs=|+-
  F : Outport
  wires:
  x/1 -> Sum/1
  x_ref/1 -> Sum/2
  Sum/1 -> PID_Cart_Position/1
  PID_Cart_Position/1 -> Sum1/1
  theta/1 -> Sum1/2
  Sum1/1 -> PID_Pendulum_Angle/1
  PID_Pendulum_Angle/1 -> F/1

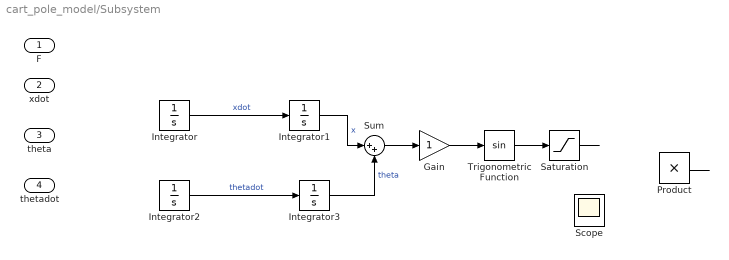
== system cart_pole_model/Subsystem ==
  F : Inport
  xdot : Inport  Port=2
  theta : Inport  Port=3
  thetadot : Inport  Port=4
  Gain : Gain
  Integrator{,1..3} (4 alike) : Integrator
  Product : Product
  Saturation : Saturate
  Scope : Scope
  Sum : Sum  Inputs=|++
  Trigonometric Function : Trigonometry
  wires:
  Trigonometric Function/1 -> Saturation/1
  Integrator/1 -> Integrator1/1  "xdot"
  Sum/1 -> Gain/1
  Integrator2/1 -> Integrator3/1  "thetadot"
  Saturation/1 -> ?
  Gain/1 -> Trigonometric Function/1
  Integrator3/1 -> Sum/2  "theta"
  Integrator1/1 -> Sum/1  "x"
  Product/1 -> ?
  ? -> Scope/1
  ? -> Integrator/1  "xddot"
  ? -> Integrator2/1  "thetaddot"

== matlab function cart_pole_model/Cart Dynamics 4/Cart Dynamics 2 ==
  data: F input; xddot output; xdot input; theta input; thetadot input; m parameter; b parameter; g parameter; M parameter; I parameter; l parameter
function xddot  = fcn(F, xdot, theta, thetadot, m, b, g, M, I, l)

    % --- Спільні члени для спрощення рівнянь ---
    A = F - b*xdot + m*(l/2)*(thetadot^2)*sin(theta);
    B = m*g*(l/2)*sin(theta);
    C = m*(l/2)*cos(theta);
    D = (M + m)*I - C^2; % Знаменник

    % --- Твої диференціальні рівняння ---
    xddot = (I*A + C*B) / D;
end

== matlab function cart_pole_model/Pendulum Dynamics 4/Pendulum Dynamics 2 ==
  data: F input; thetaddot output; xdot input; theta input; thetadot input; m parameter; M parameter; b parameter; g parameter; I parameter; l parameter
function thetaddot  = fcn(F, xdot, theta, thetadot, m, M, b, g, I, l)

    % --- Спільні члени для спрощення рівнянь ---
    A = F - b*xdot + m*(l/2)*(thetadot^2)*sin(theta);
    B = m*g*(l/2)*sin(theta);
    C = m*(l/2)*cos(theta);
    D = (M + m)*I - C^2; % Знаменник

    % --- Твої диференціальні рівняння ---
    thetaddot = (-C*A + (M + m)*B) / D;
end

== matlab function cart_pole_model/Cart Dynamics 2/Cart Dynamics 2 ==
  data: F input; xddot output; xdot input; theta input; thetadot input
function xddot  = fcn(F, xdot, theta, thetadot)
    % --- Параметри системи (впиши свої значення) ---
    M = 1.0;    % Маса візка (M)
    m = 0.2;    % Маса маятника (m)
    l = 1.0;    % Довжина маятника (l)
    g = 9.81;   % Прискорення вільного падіння (g)
    I = (1/12)*m*l^2;  % Момент інерції маятника (I)
    b = 0.1;    % Коефіцієнт тертя візка (b)

    % --- Спільні члени для спрощення рівнянь ---
    A = F - b*xdot + m*(l/2)*(thetadot^2)*sin(theta);
    B = m*g*(l/2)*sin(theta);
    C = m*(l/2)*cos(theta);
    D = (M + m)*I - C^2; % Знаменник

    % --- Твої диференціальні рівняння ---
    xddot = (I*A + C*B) / D;
end

== matlab function cart_pole_model/Pendulum Cart Dynamics ==
  data: F input; xddot output; xdot input; theta input; thetadot input; thetaddot output
function [xddot, thetaddot] = fcn(F, xdot, theta, thetadot)
    % --- Параметри системи (впиши свої значення) ---
    M = 1.0;    % Маса візка (M)
    m = 0.2;    % Маса маятника (m)
    l = 1.0;    % Довжина маятника (l)
    g = 9.81;   % Прискорення вільного падіння (g)
    I = (1/12)*m*l^2;  % Момент інерції маятника (I)
    b = 0.1;    % Коефіцієнт тертя візка (b)

    % --- Спільні члени для спрощення рівнянь ---
    A = F - b*xdot + m*(l/2)*(thetadot^2)*sin(theta);
    B = m*g*(l/2)*sin(theta);
    C = m*(l/2)*cos(theta);
    D = (M + m)*I - C^2; % Знаменник

    % --- Твої диференціальні рівняння ---
    xddot = (I*A + C*B) / D;
    thetaddot = (-C*A + (M + m)*B) / D;
end

== matlab function cart_pole_model/Pendulum Dynamics 2/Pendulum Dynamics 2 ==
  data: F input; thetaddot output; xdot input; theta input; thetadot input
function thetaddot  = fcn(F, xdot, theta, thetadot)
    % --- Параметри системи (впиши свої значення) ---
    M = 1.0;    % Маса візка (M)
    m = 0.2;    % Маса маятника (m)
    l = 1.0;    % Довжина маятника (l)
    g = 9.81;   % Прискорення вільного падіння (g)
    I = (1/12)*m*l^2;  % Момент інерції маятника (I)
    b = 0.1;    % Коефіцієнт тертя візка (b)

    % --- Спільні члени для спрощення рівнянь ---
    A = F - b*xdot + m*(l/2)*(thetadot^2)*sin(theta);
    B = m*g*(l/2)*sin(theta);
    C = m*(l/2)*cos(theta);
    D = (M + m)*I - C^2; % Знаменник

    % --- Твої диференціальні рівняння ---
    thetaddot = (-C*A + (M + m)*B) / D;
end

== matlab function cart_pole_model/Cart Dynamics 3/Cart Dynamics 2 ==
  data: F input; xddot output; xdot input; theta input; thetadot input; m parameter; b parameter; g parameter; M parameter; I parameter; l parameter
function xddot  = fcn(F, xdot, theta, thetadot, m, b, g, M, I, l)

    % --- Спільні члени для спрощення рівнянь ---
    A = F - b*xdot + m*(l/2)*(thetadot^2)*sin(theta);
    B = m*g*(l/2)*sin(theta);
    C = m*(l/2)*cos(theta);
    D = (M + m)*I - C^2; % Знаменник

    % --- Твої диференціальні рівняння ---
    xddot = (I*A + C*B) / D;
end

== matlab function cart_pole_model/Pendulum Dynamics 3/Pendulum Dynamics 2 ==
  data: F input; thetaddot output; xdot input; theta input; thetadot input; m parameter; M parameter; b parameter; g parameter; I parameter; l parameter
function thetaddot  = fcn(F, xdot, theta, thetadot, m, M, b, g, I, l)

    % --- Спільні члени для спрощення рівнянь ---
    A = F - b*xdot + m*(l/2)*(thetadot^2)*sin(theta);
    B = m*g*(l/2)*sin(theta);
    C = m*(l/2)*cos(theta);
    D = (M + m)*I - C^2; % Знаменник

    % --- Твої диференціальні рівняння ---
    thetaddot = (-C*A + (M + m)*B) / D;
end

== matlab function cart_pole_model/Cart Dynamics 1/Cart Dynamics 2 ==
  data: F input; xddot output; xdot input; theta input; thetadot input; m parameter; b parameter; g parameter; M parameter; I parameter; l parameter
function xddot  = fcn(F, xdot, theta, thetadot, m, b, g, M, I, l)

    % --- Спільні члени для спрощення рівнянь ---
    A = F - b*xdot + m*(l/2)*(thetadot^2)*sin(theta);
    B = m*g*(l/2)*sin(theta);
    C = m*(l/2)*cos(theta);
    D = (M + m)*I - C^2; % Знаменник

    % --- Твої диференціальні рівняння ---
    xddot = (I*A + C*B) / D;
end

== matlab function cart_pole_model/Pendulum Dynamics 1/Pendulum Dynamics 2 ==
  data: F input; thetaddot output; xdot input; theta input; thetadot input; m parameter; M parameter; b parameter; g parameter; I parameter; l parameter
function thetaddot  = fcn(F, xdot, theta, thetadot, m, M, b, g, I, l)

    % --- Спільні члени для спрощення рівнянь ---
    A = F - b*xdot + m*(l/2)*(thetadot^2)*sin(theta);
    B = m*g*(l/2)*sin(theta);
    C = m*(l/2)*cos(theta);
    D = (M + m)*I - C^2; % Знаменник

    % --- Твої диференціальні рівняння ---
    thetaddot = (-C*A + (M + m)*B) / D;
end
